simulink model "simL0_multiPath"  (R2024a)
settings: Solver=ode4  StartTime=0.0  StopTime=1500  FixedStep=0.01  MaxStep=0.01  MinStep=10^-3  RelTol=0.01
values from neighbouring files (symbols this model uses):
  MegAWESkite = yaml.ReadYaml('MegAWESkite.yaml',false,true)    [runMain.m]
undefined symbols (not defined in the file or in its folder): actuatorLimit, controllerGains_retraction, controllerGains_traction, DiscIntNeverNeededParam, ENVMT, pathparam, simInit, tetherParams, winchParameter
libraries: simulink x9, slpidlib x9, sharedtransform x3, aerolibutil x3, dspswit3 x2, dspinverses x2, shared6dof x1, simulink_extras x1, dspsigops x1, dspstat3 x1, vrlib x1
(part 2 of 5)

== system simL0_multiPath/GroundStationMegAWES/PureTorqueControl ==
  F_t_m_grnd : Inport
  F_t_set : Inport  Port=2
  theta_dot : Inport  Port=3
  Enable : EnablePort  StatesWhenEnabling=reset
  Constant4 : Constant  Value=winchParameter.a_max/winchParameter.radius
  Constant5 : Constant  Value=winchParameter.a_min/winchParameter.radius
  Dot Product1 : DotProduct  OutDataTypeStr=Inherit: Inherit via internal rule
  FT set : Scope  NumInputPorts=2
  Gain : Gain  Gain=winchParameter.inertia
  Gain1 : Gain  Gain=winchParameter.inertia
  Gain2 : Gain  Gain=winchParameter.friction
  Gain4 : Gain  Gain=winchParameter.radius
  PID Controller : slpidlib/PID Controller  Controller=PI  Form=Parallel  TimeDomain=Continuous-time  UseExternalTs=off  SampleTime=-1  IntegratorMethod=Forward Euler  FilterMethod=Forward Euler  ControllerParametersSource=internal  P=winchParameter.kp  I=winchParameter.ki  UseKiTs=off  D=0  UseExternalDerivativeSource=off  N=100  UseFilter=on  TunerSelectOption=Transfer Function Based (PID Tuner App)  InitialConditionSource=internal  InitialConditionForIntegrator=0  InitialConditionForFilter=0  DifferentiatorICPrevScaledInput=0  ExternalReset=none  TrackingMode=off  Kt=1  LimitOutput=off  SatLimitsSource=internal  UpperSaturationLimit=inf  LowerSaturationLimit=-inf  LinearizeAsGain=on  AntiWindupMode=none  Kb=1  LimitIntegrator=off  UpperIntegratorSaturationLimit=inf  LowerIntegratorSaturationLimit=-inf  POutMin=[]  POutMax=[]  IOutMin=[]  IOutMax=[]  DOutMin=[]  DOutMax=[]  NOutMin=[]  NOutMax=[]  SumOutMin=[]  SumOutMax=[]  SaturationOutMin=[]  SaturationOutMax=[]  PParamMin=[]  PParamMax=[]  IParamMin=[]  IParamMax=[]  DParamMin=[]  DParamMax=[]  NParamMin=[]  NParamMax=[]  KbParamMin=[]  KbParamMax=[]  KtParamMin=[]  KtParamMax=[]  KbOutMin=[]  KbOutMax=[]  KtOutMin=[]  KtOutMax=[]  IntegratorOutMin=[]  IntegratorOutMax=[]  FilterOutMin=[]  FilterOutMax=[]  SumI1OutMin=[]  SumI1OutMax=[]  SumI2OutMin=[]  SumI2OutMax=[]  SumI3OutMin=[]  SumI3OutMax=[]  SumI4OutMin=[]  SumI4OutMax=[]  SumDOutMin=[]  SumDOutMax=[]  DifferentiatorOutMin=[]  DifferentiatorOutMax=[]  FilterDiffOutCoefMin=[]  FilterDiffOutCoefMax=[]  ReciprocalOutMin=[]  ReciprocalOutMax=[]  SumDenOutMin=[]  SumDenOutMax=[]  SumNumOutMin=[]  SumNumOutMax=[]  DivideOutMin=[]  DivideOutMax=[]  UdiffTsProdOutMin=[]  UdiffTsProdOutMax=[]  NTsProdOutMin=[]  NTsProdOutMax=[]  UintegralTsProdOutMin=[]  UintegralTsProdOutMax=[]  UngainTsProdOutMin=[]  UngainTsProdOutMax=[]  ClampingZeroOutDataTypeStr=Inherit: Inherit via back propagation  ClampingZeroOutMin=[]  ClampingZeroOutMax=[]  FilterDenConstantOutDataTypeStr=Inherit: Inherit via back propagation  FilterDenConstantOutMin=[]  FilterDenConstantOutMax=[]  PCopyOutDataTypeStr=Inherit: Inherit via back propagation  PCopyOutMin=[]  PCopyOutMax=[]  NCopyOutDataTypeStr=Inherit: Inherit via back propagation  NCopyOutMin=[]  NCopyOutMax=[]  IntegratorContinuousStateAttributes=''  IntegratorStateMustResolveToSignalObject=off  IntegratorRTWStateStorageClass=Auto  FilterContinuousStateAttributes=''  FilterStateMustResolveToSignalObject=off  FilterRTWStateStorageClass=Auto  ParallelPVariant=InternalParameters  IdealPVariant=Disabled  IVariant=InternalParameters  DVariant=Disabled  IntegratorVariant=Continuous  SatVariant=Disabled  AWVariant=Passthrough  PCopyVariant=Disabled  TRVariant=Disabled  FdbkBlocksVariant=Forward  IdealPFdbkVariant=Disabled  SatFdbkVariant=Disabled  DerivativeFilterVariant=Disabled  NVariant=Disabled  NCopyVariant=Disabled_SignalSpec  FilterICVariant=Disabled  IntegratorICVariant=InternalICs  ExternalResetVariant=Disabled  TRSumVariant=Passthrough  SumFdbkVariant=Disabled  SumVariant=Sum_PI  TsampFilterVariant=InternalTs  TsampNgainVariant=Passthrough  TsampIntegralVariant=Disabled_SignalSpec  ExternalSaturationOutDataTypeStr=Inherit: Same as second input  DerivativeSourceVariant=Disabled
  Saturation Dynamic : simulink/Discontinuities/Saturation Dynamic  OutMin=[]  OutMax=[]  OutDataTypeStr=Inherit: Same as second input  OutDataType=fixdt(1, 16)  OutScaling=2^-10  DoSatur=off
  Sqrt1 : Sqrt
  Sum2 : Sum  Inputs=-++
  Sum4 : Sum  Inputs=-++
  Sum6 : Sum  Inputs=|-+
  torque_cmd : Outport  VectorParamsAs1DForOutWhenUnconnected=off
  wires:
  Sqrt1/1 -> FT set/1, Sum6/2
  F_t_set/1 -> FT set/2, Sum6/1
  Gain4/1 -> Sum2/1, Sum4/1
  Constant4/1 -> Gain/1
  Gain/1 -> Sum2/2
  Sum2/1 -> Saturation Dynamic/1
  Constant5/1 -> Gain1/1
  Gain1/1 -> Sum4/2
  Sum4/1 -> Saturation Dynamic/3
  Gain2/1 -> Sum4/3, Sum2/3
  Dot Product1/1 -> Sqrt1/1
  F_t_m_grnd/1 -> Dot Product1/1, Dot Product1/2, Gain4/1
  theta_dot/1 -> Gain2/1
  Sum6/1 -> PID Controller/1
  Saturation Dynamic/1 -> torque_cmd/1
  PID Controller/1 -> Saturation Dynamic/2

== system simL0_multiPath/GroundStationMegAWES/Traction winch controller ==
  v_ro : Inport
  Ft_ground_W : Inport  Port=2
  Calculate Ft_ref : Subsystem
  MegAWES convention is that a positive torque leads to reel-out : Gain  Gain=-1
  Sum : Sum  Inputs=|+-
  feedforward : Gain  Gain=winchParameter.radius
  reel-out : Scope
  tether force : Scope  NumInputPorts=3
  torque : Scope
  traction_torque_cmd : Outport
  Ft_ref : Outport  Port=2
  Ft_ground : Outport  Port=3
  wires:
  v_ro/1 -> reel-out/1, Calculate Ft_ref/1(v_ro)
  Ft_ground_W/1 -> Ft_ground/1, Sum/2, tether force/2
  Sum/1 -> tether force/3
  feedforward/1 -> MegAWES convention is that a positive torque leads to reel-out/1, torque/1  "torque_md_tot"
  MegAWES convention is that a positive torque leads to reel-out/1 -> traction_torque_cmd/1
  Calculate Ft_ref/1(Ft_ref) -> feedforward/1, Ft_ref/1, tether force/1, Sum/1

== system simL0_multiPath/GroundStationMegAWES/WinchDynamics ==
  for_tether_tot : Inport
  control_moments : Inport  Port=2
  Discrete-Time Integrator : DiscreteIntegrator  InitialCondition=winchParameter.lj_dot_init  SampleTime=-1  LimitOutput=on  UpperSaturationLimit=winchParameter.v_max/winchParameter.radius  LowerSaturationLimit=winchParameter.v_min/winchParameter.radius  ICPrevOutput=DiscIntNeverNeededParam  ICPrevScaledInput=DiscIntNeverNeededParam
  Gain{,2..6} (6 alike) : Gain  Gain=winchParameter.radius
  Gain1 : Gain  Gain=1/winchParameter.inertia
  Gain7 : Gain  Gain=winchParameter.friction
  Integrator : Integrator  InitialCondition=tetherParams.tether_inital_lenght/winchParameter.radius
  Saturation1 : Saturate  UpperLimit=winchParameter.a_max/winchParameter.radius  LowerLimit=winchParameter.a_min/winchParameter.radius
  Sum : Sum  Inputs=+-+
  winch acc : Scope  NumInputPorts=2
  tether_length : Outport  VectorParamsAs1DForOutWhenUnconnected=off
  theta_dot : Outport  Port=2  VectorParamsAs1DForOutWhenUnconnected=off
  winch_acc : Outport  Port=3  VectorParamsAs1DForOutWhenUnconnected=off
  winch_vel : Outport  Port=4  VectorParamsAs1DForOutWhenUnconnected=off
  wires:
  Gain/1 -> tether_length/1
  Gain2/1 -> Sum/1
  Sum/1 -> Gain1/1
  Integrator/1 -> Gain/1  "winch_angle"
  Discrete-Time Integrator/1 -> Gain4/1, Gain7/1, theta_dot/1, Integrator/1  "winch_angVel"
  control_moments/1 -> Sum/3
  Gain7/1 -> Sum/2
  for_tether_tot/1 -> Gain2/1
  Gain1/1 -> Saturation1/1, Gain5/1, Gain3/1
  Saturation1/1 -> Discrete-Time Integrator/1, Gain6/1  "omega_dot"
  Gain4/1 -> winch_vel/1
  Gain3/1 -> winch_acc/1
  Gain5/1 -> winch acc/1
  Gain6/1 -> winch acc/2

== system simL0_multiPath/Output/Convergence_check ==
  P_mech : Inport
  flightMode : Inport  Port=2
  AND : Logic  AllPortsSameDT=off  OutDataTypeStr=boolean
  Compare To Constant1 : simulink/Logic and Bit Operations/Compare To Constant  relop=>=  const=simInit.numCyclesMinimumConv  OutDataTypeStr=boolean
  Constant1 : Constant  Value=simInit.thresholdConv_power/simInit.numCyclesMinimumConv
  Delay{1..4,6..7} (6 alike) : Delay  DelayLength=1  InitialCondition=0
  Delay5 : Delay  DelayLength=1  InitialCondition=simInit.thresholdConv_power+1000
  MATLAB Function2 : MATLAB Function  TreatAsAtomicUnit=on
  Matrix Multiply : Product
  Relational Operator1 : RelationalOperator  Operator=<=  OutDataTypeStr=boolean  RndMeth=Simplest  InputSameDT=off
  Scope : Scope
  Scope1 : Scope
  Stop Simulation : Stop
  power_conv_flag : Outport  VectorParamsAs1DForOutWhenUnconnected=off
  error_power : Outport  Port=2  VectorParamsAs1DForOutWhenUnconnected=off
  No_cycles : Outport  Port=3
  cycle_signal_counter : Outport  Port=4  VectorParamsAs1DForOutWhenUnconnected=off
  wires:
  Delay5/1 -> MATLAB Function2/7(e_old)
  Constant1/1 -> Matrix Multiply/1
  Matrix Multiply/1 -> Relational Operator1/2
  Compare To Constant1/1 -> AND/2
  flightMode/1 -> Scope1/1, MATLAB Function2/6(flightMode)
  Delay7/1 -> MATLAB Function2/8("cnt_max_mat ")
  MATLAB Function2/4(cnt) -> Delay1/1
  Delay4/1 -> MATLAB Function2/1("flag ")
  Delay3/1 -> MATLAB Function2/3("p_sum ")
  Relational Operator1/1 -> AND/1
  Delay1/1 -> MATLAB Function2/4("cnt ")
  MATLAB Function2/3(p_sum) -> Delay3/1
  MATLAB Function2/1(flag) -> Delay4/1
  Delay2/1 -> MATLAB Function2/2(m_old)
  MATLAB Function2/7(cycles_cnt) -> Delay6/1, No_cycles/1, Matrix Multiply/2, Compare To Constant1/1, Scope/1
  MATLAB Function2/2(m_new) -> Delay2/1
  AND/1 -> power_conv_flag/1, Stop Simulation/1
  P_mech/1 -> MATLAB Function2/5(u)
  Delay6/1 -> MATLAB Function2/9("cycles_cnt ")
  MATLAB Function2/6(cnt_max_mat) -> cycle_signal_counter/1, Delay7/1
  MATLAB Function2/5(e_new) -> Delay5/1, error_power/1, Relational Operator1/1

== system simL0_multiPath/aerodynamic forces/HLW ==
  In1 : Inport
  Switch Solver Compiled : MATLAB Function  TreatAsAtomicUnit=on
  Out1 : Outport  VectorParamsAs1DForOutWhenUnconnected=off
  wires:
  Switch Solver Compiled/1(out) -> Out1/1
  In1/1 -> Switch Solver Compiled/1(input)

== system simL0_multiPath/aerodynamic forces/Lookup Tables ==
  Inputs : Inport
  Switch Solver Compiled : MATLAB Function  TreatAsAtomicUnit=on
  ForceMoment : Outport  VectorParamsAs1DForOutWhenUnconnected=off
  wires:
  Switch Solver Compiled/1(out) -> ForceMoment/1
  Inputs/1 -> Switch Solver Compiled/1(input)

== system simL0_multiPath/aerodynamic forces/SLW ==
  In1 : Inport
  Switch Solver Compiled : MATLAB Function  TreatAsAtomicUnit=on
  Out1 : Outport  VectorParamsAs1DForOutWhenUnconnected=off
  wires:
  Switch Solver Compiled/1(out) -> Out1/1
  In1/1 -> Switch Solver Compiled/1(input)

== system simL0_multiPath/aerodynamic forces/Subsystem ==
  In1 : Inport
  Demux5 : Demux  Outputs=10
  Mux : Mux  Inputs=8
  Mux1 : Mux  Inputs=2
  Out1 : Outport  VectorParamsAs1DForOutWhenUnconnected=off
  Out2 : Outport  Port=2  VectorParamsAs1DForOutWhenUnconnected=off
  wires:
  Demux5/3 -> Mux/3
  Demux5/7 -> Mux/7
  In1/1 -> Demux5/1
  Demux5/1 -> Mux/1
  Demux5/4 -> Mux/4
  Mux/1 -> Out1/1
  Demux5/5 -> Mux/5
  Demux5/6 -> Mux/6
  Demux5/8 -> Mux/8
  Demux5/9 -> Mux1/1
  Demux5/2 -> Mux/2
  Demux5/10 -> Mux1/2
  Mux1/1 -> Out2/1

== system simL0_multiPath/aerodynamic forces/Subsystem1 ==
  note: OLD
  note: increases the flap angle on the side, towards which the plane is rolling
  In1 : Inport
  Gain1 : Gain  Commented=on  Gain=-1.5
  Gain2 : Gain  Commented=on  Gain=-1
  Gain4 : Gain  Commented=on
  Gain5 : Gain  Commented=on  Gain=1.5
  Gain6 : Gain  Gain=-1
  Gain7 : Gain
  Switch : Switch  Commented=on  Criteria=u2 > Threshold  SaturateOnIntegerOverflow=off  InputSameDT=off
  Switch1 : Switch  Commented=on  Criteria=u2 > Threshold  SaturateOnIntegerOverflow=off  InputSameDT=off
  left flap : Outport  VectorParamsAs1DForOutWhenUnconnected=off
  right flap : Outport  Port=2  VectorParamsAs1DForOutWhenUnconnected=off
  wires:
  Gain1/1 -> Switch/1
  Gain2/1 -> Switch/3
  Gain4/1 -> Switch1/1
  Gain5/1 -> Switch1/3
  Gain6/1 -> right flap/1
  Gain7/1 -> left flap/1
  In1/1 -> Gain4/1, Switch1/2, Gain5/1, Gain2/1, Switch/2, Gain1/1, Gain6/1, Gain7/1

== system simL0_multiPath/Controls/ FlightControl/Angle_of_Attack ==
  desired_descent_angle : Inport
  flightState : Inport  Port=2
  Constant12 : Constant  Value=MegAWESkite.MainWing.alphaMax
  Degrees to Radians : simulink_extras/Transformations/Degrees to Radians
  Multiply : Gain  Gain=0.75
  Multiport Switch3 : MultiPortSwitch  DiagnosticForDefault=None  SaturateOnIntegerOverflow=off  InputSameDT=off
  desired_alpha : Outport
  wires:
  desired_descent_angle/1 -> Multiport Switch3/4, Multiport Switch3/3
  Degrees to Radians/1 -> Multiport Switch3/2
  flightState/1 -> Multiport Switch3/1
  Constant12/1 -> Multiply/1
  Multiply/1 -> Degrees to Radians/1
  Multiport Switch3/1 -> desired_alpha/1

== system simL0_multiPath/Controls/ FlightControl/Convert YPR-e_to_tan ==
  kite_pos : Inport
  kite_angles : Inport  Port=2
  Convert YPR-etotan : MATLAB Function  TreatAsAtomicUnit=on
  Demux8 : Demux  Outputs=3
  Demux9 : Demux  Outputs=3
  Mux5 : Mux  Inputs=6
  Scope15 : Scope
  roll_tang : Outport
  pitch_tang : Outport  Port=2
  yaw_tang : Outport  Port=3
  actual_roll : Outport  Port=4
  wires:
  Demux8/2 -> Mux5/2
  Demux9/3 -> Mux5/6
  Convert YPR-etotan/2(a_pitch) -> pitch_tang/1
  Demux8/3 -> Mux5/3
  Demux9/2 -> Mux5/5
  Convert YPR-etotan/1(a_roll) -> Scope15/1, roll_tang/1
  Convert YPR-etotan/3(a_yaw) -> yaw_tang/1
  Demux8/1 -> Mux5/1
  Mux5/1 -> Convert YPR-etotan/1(input)
  kite_angles/1 -> Demux9/1
  Demux9/1 -> actual_roll/1, Mux5/4
  kite_pos/1 -> Demux8/1

== system simL0_multiPath/Controls/ FlightControl/EarthtoWind ==
  E_vec : Inport
  Demux : Demux  Outputs=3
  Gain : Gain
  Gain1 : Gain  Gain=-1
  Gain2 : Gain  Gain=-1
  Mux4 : Mux  Inputs=3
  W_vec : Outport
  wires:
  Demux/2 -> Gain1/1
  Demux/1 -> Gain/1
  Gain1/1 -> Mux4/2
  Gain/1 -> Mux4/1
  Gain2/1 -> Mux4/3
  E_vec/1 -> Demux/1
  Mux4/1 -> W_vec/1
  Demux/3 -> Gain2/1

== system simL0_multiPath/Controls/ FlightControl/EarthtoWind1 ==
  E_vec : Inport
  Demux : Demux  Outputs=3
  Gain : Gain
  Gain1 : Gain  Gain=-1
  Gain2 : Gain  Gain=-1
  Mux4 : Mux  Inputs=3
  W_vec : Outport
  wires:
  Demux/2 -> Gain1/1
  Demux/1 -> Gain/1
  Gain1/1 -> Mux4/2
  Gain/1 -> Mux4/1
  Gain2/1 -> Mux4/3
  E_vec/1 -> Demux/1
  Mux4/1 -> W_vec/1
  Demux/3 -> Gain2/1

== system simL0_multiPath/Controls/ FlightControl/EarthtoWind2 ==
  E_vec : Inport
  Demux : Demux  Outputs=3
  Gain : Gain
  Gain1 : Gain  Gain=-1
  Gain2 : Gain  Gain=-1
  Mux4 : Mux  Inputs=3
  W_vec : Outport
  wires:
  Demux/2 -> Gain1/1
  Demux/1 -> Gain/1
  Gain1/1 -> Mux4/2
  Gain/1 -> Mux4/1
  Gain2/1 -> Mux4/3
  E_vec/1 -> Demux/1
  Mux4/1 -> W_vec/1
  Demux/3 -> Gain2/1

== system simL0_multiPath/Controls/ FlightControl/EarthtoWind3 ==
  E_vec : Inport
  Demux : Demux  Outputs=3
  Gain : Gain
  Gain1 : Gain  Gain=-1
  Gain2 : Gain  Gain=-1
  Mux4 : Mux  Inputs=3
  W_vec : Outport
  wires:
  Demux/2 -> Gain1/1
  Demux/1 -> Gain/1
  Gain1/1 -> Mux4/2
  Gain/1 -> Mux4/1
  Gain2/1 -> Mux4/3
  E_vec/1 -> Demux/1
  Mux4/1 -> W_vec/1
  Demux/3 -> Gain2/1

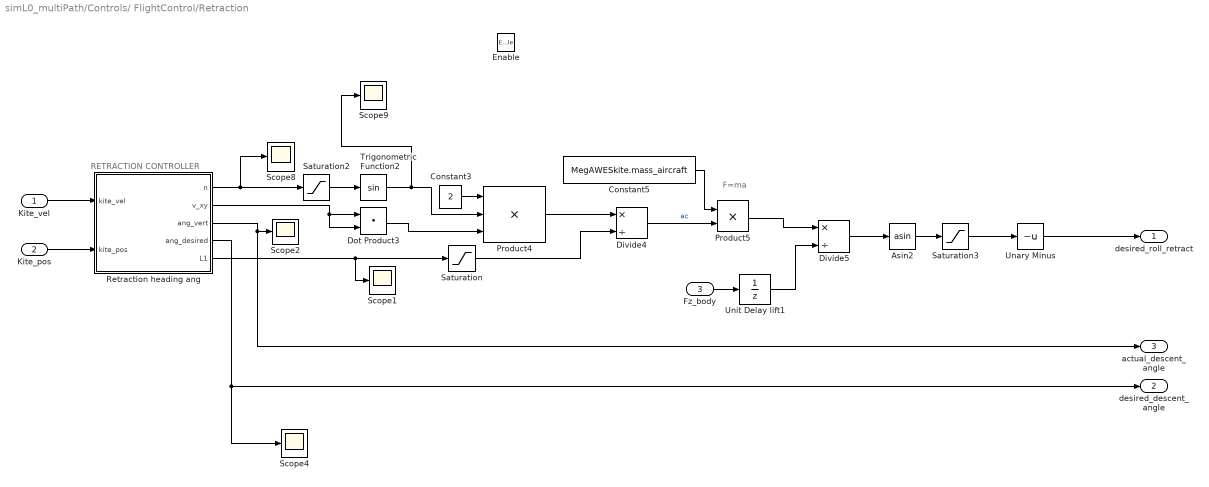
== system simL0_multiPath/Controls/ FlightControl/Retraction ==
  note: F=ma
  note: RETRACTION CONTROLLER
  Kite_vel : Inport
  Kite_pos : Inport  Port=2
  Fz_body : Inport  Port=3
  Enable : EnablePort  StatesWhenEnabling=reset
  Asin2 : Trigonometry  Operator=asin
  Constant3 : Constant  Value=2
  Constant5 : Constant  Value=MegAWESkite.mass_aircraft
  Divide4 : Product  Inputs=*/
  Divide5 : Product  Inputs=*/
  Dot Product3 : DotProduct  OutDataTypeStr=Inherit: Inherit via internal rule
  Product4 : Product  Inputs=3
  Product5 : Product
  Retraction heading ang : MATLAB Function  TreatAsAtomicUnit=on
  Saturation : Saturate  UpperLimit=inf  LowerLimit=100
  Saturation2 : Saturate  UpperLimit=pi/2  LowerLimit=-pi/2
  Saturation3 : Saturate  UpperLimit=1  LowerLimit=-1
  Scope{1..2,4,8..9} (5 alike) : Scope
  Trigonometric Function2 : Trigonometry
  Unary Minus : UnaryMinus
  Unit Delay lift1 : UnitDelay  InitialCondition=1  SampleTime=-1  HasFrameUpgradeWarning=on
  desired_roll_retract : Outport
  desired_descent_angle : Outport  Port=2
  actual_descent_angle : Outport  Port=3
  wires:
  Saturation3/1 -> Unary Minus/1
  Retraction heading ang/3(ang_vert) -> actual_descent_angle/1, Scope2/1
  Retraction heading ang/1(n) -> Scope8/1, Saturation2/1
  Fz_body/1 -> Unit Delay lift1/1
  Product4/1 -> Divide4/1
  Retraction heading ang/2(v_xy) -> Dot Product3/2, Dot Product3/1
  Divide4/1 -> Product5/2  "ac"
  Retraction heading ang/4(ang_desired) -> desired_descent_angle/1, Scope4/1
  Unary Minus/1 -> desired_roll_retract/1
  Divide5/1 -> Asin2/1
  Constant3/1 -> Product4/1
  Dot Product3/1 -> Product4/3
  Kite_vel/1 -> Retraction heading ang/1(kite_vel)
  Asin2/1 -> Saturation3/1
  Trigonometric Function2/1 -> Scope9/1, Product4/2
  Kite_pos/1 -> Retraction heading ang/2(kite_pos)
  Product5/1 -> Divide5/1
  Unit Delay lift1/1 -> Divide5/2
  Saturation2/1 -> Trigonometric Function2/1
  Constant5/1 -> Product5/1
  Retraction heading ang/5(L1) -> Scope1/1, Saturation/1
  Saturation/1 -> Divide4/2

== system simL0_multiPath/Controls/ FlightControl/Switch_flystate ==
  s_path : Inport
  Counter1 : dspswit3/Counter  Direction=Up  CountEvent=Rising edge  CounterSize=User defined  MaxCount=255  InitialCount=0  Output=Count  HitValue=32  ResetInput=off  SamplesPerFrame=1  Ts=1  CntDtype=double  HitDtype=Logical
  MATLAB Function : MATLAB Function  TreatAsAtomicUnit=on
  Zero Crossing : dspsigops/Zero Crossing  InputProcessing=Columns as channels (frame based)
  n_cycle : Outport
  pos_cond : Outport  Port=2
  trans_flag : Outport  Port=3
  wires:
  Counter1/1 -> n_cycle/1
  s_path/1 -> MATLAB Function/1(s)
  Zero Crossing/1 -> Counter1/1
  MATLAB Function/1(r) -> pos_cond/1, Zero Crossing/1
  MATLAB Function/2(t) -> trans_flag/1

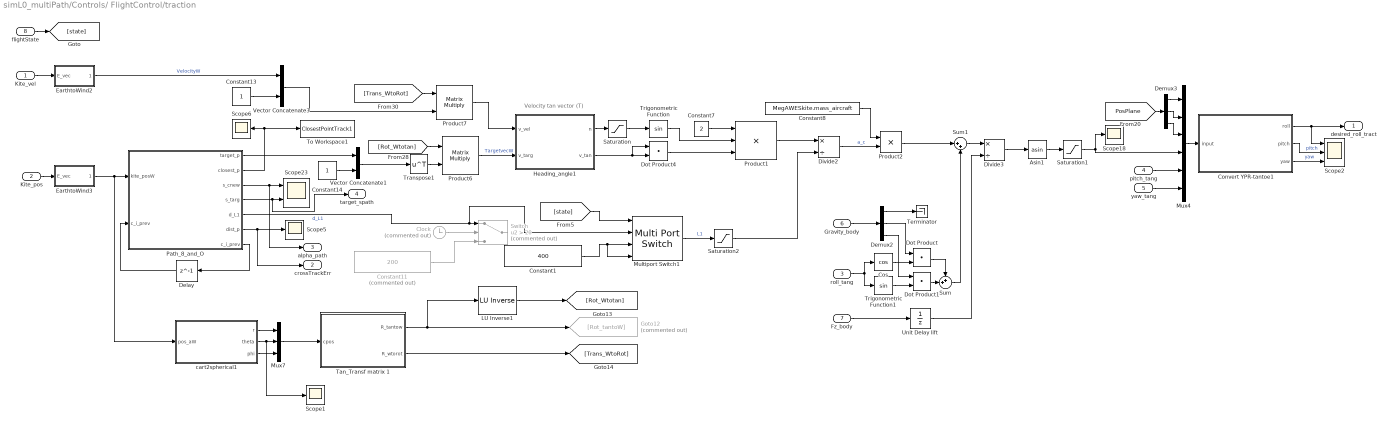
== system simL0_multiPath/Controls/ FlightControl/traction ==
  note: Velocity tan vector (T)
  Kite_vel : Inport
  Kite_pos : Inport  Port=2
  roll_tang : Inport  Port=3
  pitch_tang : Inport  Port=4
  yaw_tang : Inport  Port=5
  Gravity_body : Inport  Port=6
  Fz_body : Inport  Port=7
  flightState : Inport  Port=8
  " LU Inverse1" : dspinverses/ LU Inverse
  Asin1 : Trigonometry  Operator=asin
  Clock : Clock  Commented=on
  Constant1 : Constant  Value=400
  Constant11 : Constant  Commented=on  Value=200
  Constant13 : Constant
  Constant14 : Constant
  Constant7 : Constant  Value=2
  Constant8 : Constant  Value=MegAWESkite.mass_aircraft
  Convert YPR-tantoe1 : MATLAB Function  TreatAsAtomicUnit=on
  Cos : Trigonometry  Operator=cos
  Delay : Delay  DelayLength=1  InitialCondition=25
  Demux2 : Demux  Outputs=3
  Demux3 : Demux  Outputs=3
  Divide2 : Product  Inputs=*/
  Divide3 : Product  Inputs=*/
  Dot Product : DotProduct  OutDataTypeStr=Inherit: Inherit via internal rule
  Dot Product1 : DotProduct  OutDataTypeStr=Inherit: Inherit via internal rule
  Dot Product4 : DotProduct  OutDataTypeStr=Inherit: Inherit via internal rule
  EarthtoWind2 : Subsystem
  EarthtoWind3 : Subsystem
  Goto12 : Goto  Commented=on  GotoTag=Rot_tantoW
  Heading_angle1 : MATLAB Function  TreatAsAtomicUnit=on
  Multiport Switch1 : MultiPortSwitch  DiagnosticForDefault=None  SaturateOnIntegerOverflow=off  InputSameDT=off
  Mux4 : Mux  Inputs=6
  Mux7 : Mux  Inputs=3
  Path_8_and_O : MATLAB Function  TreatAsAtomicUnit=on
  Product1 : Product  Inputs=3
  Product2 : Product
  Product6 : Product  Multiplication=Matrix(*)
  Product7 : Product  Multiplication=Matrix(*)
  Saturation : Saturate  UpperLimit=pi/4  LowerLimit=-pi/4
  Saturation1 : Saturate  UpperLimit=1  LowerLimit=-1
  Saturation2 : Saturate  UpperLimit=inf  LowerLimit=50
  Scope{1,5..6,18} (4 alike) : Scope
  Scope2 : Scope  NumInputPorts=3
  Scope23 : Scope  NumInputPorts=2
  Sum : Sum  Inputs=++|
  Sum1 : Sum  Inputs=|++
  Switch : Switch  Commented=on  Criteria=u2 > Threshold  Threshold=20  SaturateOnIntegerOverflow=off  InputSameDT=off
  Tan_Transf matrix 1 : MATLAB Function  TreatAsAtomicUnit=on
  Terminator : Terminator
  To Workspace1 : ToWorkspace  VariableName=ClosestPointTrack1  SaveFormat=Timeseries  SampleTime=-1
  Transpose1 : Math  Operator=transpose
  Trigonometric Function : Trigonometry
  Trigonometric Function1 : Trigonometry
  Unit Delay lift : UnitDelay  InitialCondition=1  SampleTime=-1  HasFrameUpgradeWarning=on
  Vector Concatenate1 : Concatenate
  Vector Concatenate3 : Concatenate
  cart2spherical1 : MATLAB Function  TreatAsAtomicUnit=on
  desired_roll_tract : Outport
  crossTrackErr : Outport  Port=2
  alpha_path : Outport  Port=3
  target_spath : Outport  Port=4
  wires:
  Demux2/3 -> Dot Product1/1
  Constant13/1 -> Vector Concatenate3/2
  Convert YPR-tantoe1/3(yaw) -> Scope2/3  "yaw"
  Heading_angle1/2(v_tan) -> Dot Product4/1, Dot Product4/2
  Dot Product/1 -> Sum/1
  Constant8/1 -> Product2/1
  Convert YPR-tantoe1/1(roll) -> desired_roll_tract/1, Scope2/1
  Trigonometric Function/1 -> Product1/2
  Path_8_and_O/3(s_cnew) -> alpha_path/1, Scope23/1
  Path_8_and_O/4(s_targ) -> target_spath/1, Scope23/2
  Product7/1 -> Heading_angle1/1(v_vel)
  Demux3/3 -> Mux4/3
  Saturation/1 -> Trigonometric Function/1
  Dot Product1/1 -> Sum/2
  Demux3/2 -> Mux4/2
  Divide2/1 -> Product2/2  "a_c"
  Product2/1 -> Sum1/1
  Cos/1 -> Dot Product/2
  Divide3/1 -> Asin1/1
  Constant7/1 -> Product1/1
  Asin1/1 -> Saturation1/1
  Gravity_body/1 -> Demux2/1
  Product1/1 -> Divide2/1
  Heading_angle1/1(n) -> Saturation/1
  Unit Delay lift/1 -> Divide3/2
  Path_8_and_O/6(dist_p) -> crossTrackErr/1, Scope5/1
  Sum/1 -> Sum1/2
  EarthtoWind2/1(W_vec) -> Vector Concatenate3/1  "VelocityW"
  Convert YPR-tantoe1/2(pitch) -> Scope2/2  "pitch"
  Saturation1/1 -> Scope18/1, Mux4/4
  [state] -> Multiport Switch1/1
  Mux4/1 -> Convert YPR-tantoe1/1(input)
  Demux3/1 -> Mux4/1
  Trigonometric Function1/1 -> Dot Product1/2
  Demux2/1 -> Terminator/1
  Fz_body/1 -> Unit Delay lift/1
  Multiport Switch1/1 -> Saturation2/1  "L1"
  Vector Concatenate3/1 -> Product7/2
  [Trans_WtoRot] -> Product7/1
  Demux2/2 -> Dot Product/1
  [PosPlane] -> Demux3/1
  pitch_tang/1 -> Mux4/5
  [Rot_Wtotan] -> Product6/1
  Constant14/1 -> Vector Concatenate1/2
  Transpose1/1 -> Product6/2
  Kite_pos/1 -> EarthtoWind3/1(E_vec)
  Product6/1 -> Heading_angle1/2(v_targ)  "TargetvecW"
  Sum1/1 -> Divide3/1
  Dot Product4/1 -> Product1/3
  Path_8_and_O/1(target_p) -> Vector Concatenate1/1
  yaw_tang/1 -> Mux4/6
  Vector Concatenate1/1 -> Transpose1/1
  Path_8_and_O/5(d_L1) -> Multiport Switch1/2, Switch/1  "d_L1"
  roll_tang/1 -> Trigonometric Function1/1, Cos/1
  Path_8_and_O/2(closest_p) -> To Workspace1/1, Scope6/1
  Kite_vel/1 -> EarthtoWind2/1(E_vec)
  " LU Inverse1"/1 -> [Rot_Wtotan]
  Mux7/1 -> Tan_Transf matrix 1/1(cpos)
  Tan_Transf matrix 1/1(R_tantow) -> Goto12/1, " LU Inverse1"/1
  cart2spherical1/1(r) -> Mux7/1
  cart2spherical1/3(phi) -> Mux7/3
  Tan_Transf matrix 1/2(R_wtorot) -> [Trans_WtoRot]
  EarthtoWind3/1(W_vec) -> cart2spherical1/1(pos_aW), Path_8_and_O/1(kite_posW)
  cart2spherical1/2(theta) -> Scope1/1, Mux7/2
  flightState/1 -> [state]
  Path_8_and_O/7(c_i_prev) -> Delay/1
  Delay/1 -> Path_8_and_O/2("c_i_prev ")
  Saturation2/1 -> Divide2/2
  Constant11/1 -> Switch/3
  Clock/1 -> Switch/2
  Constant1/1 -> Multiport Switch1/4, Multiport Switch1/3

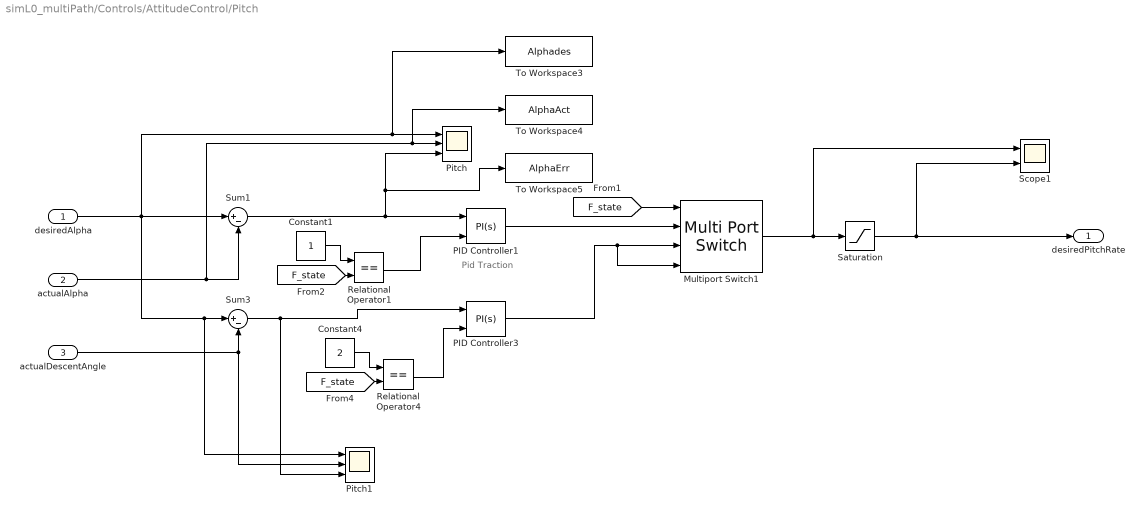
== system simL0_multiPath/Controls/AttitudeControl/Pitch ==
  note: Pid Traction
  desiredAlpha : Inport
  actualAlpha : Inport  Port=2
  actualDescentAngle : Inport  Port=3
  Constant1 : Constant
  Constant4 : Constant  Value=2
  Multiport Switch1 : MultiPortSwitch  DiagnosticForDefault=None  SaturateOnIntegerOverflow=off  InputSameDT=off
  PID Controller1 : slpidlib/PID Controller  Controller=PI  Form=Parallel  TimeDomain=Continuous-time  UseExternalTs=off  SampleTime=-1  IntegratorMethod=Forward Euler  FilterMethod=Forward Euler  ControllerParametersSource=internal  P=controllerGains_traction.attitudePitch_P  I=controllerGains_traction.attitudePitch_I  UseKiTs=off  D=0  UseExternalDerivativeSource=off  N=1  UseFilter=on  TunerSelectOption=Transfer Function Based (PID Tuner App)  InitialConditionSource=internal  InitialConditionForIntegrator=0  InitialConditionForFilter=0  DifferentiatorICPrevScaledInput=0  ExternalReset=rising  TrackingMode=off  Kt=1  LimitOutput=off  SatLimitsSource=internal  UpperSaturationLimit=pi  LowerSaturationLimit=-pi  LinearizeAsGain=on  AntiWindupMode=none  Kb=50  LimitIntegrator=off  UpperIntegratorSaturationLimit=inf  LowerIntegratorSaturationLimit=-inf  POutMin=[]  POutMax=[]  IOutMin=[]  IOutMax=[]  DOutMin=[]  DOutMax=[]  NOutMin=[]  NOutMax=[]  SumOutMin=[]  SumOutMax=[]  SaturationOutMin=[]  SaturationOutMax=[]  PParamMin=[]  PParamMax=[]  IParamMin=[]  IParamMax=[]  DParamMin=[]  DParamMax=[]  NParamMin=[]  NParamMax=[]  KbParamMin=[]  KbParamMax=[]  KtParamMin=[]  KtParamMax=[]  KbOutMin=[]  KbOutMax=[]  KtOutMin=[]  KtOutMax=[]  IntegratorOutMin=[]  IntegratorOutMax=[]  FilterOutMin=[]  FilterOutMax=[]  SumI1OutMin=[]  SumI1OutMax=[]  SumI2OutMin=[]  SumI2OutMax=[]  SumI3OutMin=[]  SumI3OutMax=[]  SumI4OutMin=[]  SumI4OutMax=[]  SumDOutMin=[]  SumDOutMax=[]  DifferentiatorOutMin=[]  DifferentiatorOutMax=[]  FilterDiffOutCoefMin=[]  FilterDiffOutCoefMax=[]  ReciprocalOutMin=[]  ReciprocalOutMax=[]  SumDenOutMin=[]  SumDenOutMax=[]  SumNumOutMin=[]  SumNumOutMax=[]  DivideOutMin=[]  DivideOutMax=[]  UdiffTsProdOutMin=[]  UdiffTsProdOutMax=[]  NTsProdOutMin=[]  NTsProdOutMax=[]  UintegralTsProdOutMin=[]  UintegralTsProdOutMax=[]  UngainTsProdOutMin=[]  UngainTsProdOutMax=[]  ClampingZeroOutDataTypeStr=Inherit: Inherit via back propagation  ClampingZeroOutMin=[]  ClampingZeroOutMax=[]  FilterDenConstantOutDataTypeStr=Inherit: Inherit via back propagation  FilterDenConstantOutMin=[]  FilterDenConstantOutMax=[]  PCopyOutDataTypeStr=Inherit: Inherit via back propagation  PCopyOutMin=[]  PCopyOutMax=[]  NCopyOutDataTypeStr=Inherit: Inherit via back propagation  NCopyOutMin=[]  NCopyOutMax=[]  IntegratorContinuousStateAttributes=''  IntegratorStateMustResolveToSignalObject=off  IntegratorRTWStateStorageClass=Auto  FilterContinuousStateAttributes=''  FilterStateMustResolveToSignalObject=off  FilterRTWStateStorageClass=Auto  ParallelPVariant=InternalParameters  IdealPVariant=Disabled  IVariant=InternalParameters  DVariant=Disabled  IntegratorVariant=Continuous  SatVariant=Disabled  AWVariant=Passthrough  PCopyVariant=Disabled  TRVariant=Disabled  FdbkBlocksVariant=Forward  IdealPFdbkVariant=Disabled  SatFdbkVariant=Disabled  DerivativeFilterVariant=Disabled  NVariant=Disabled  NCopyVariant=Disabled_SignalSpec  FilterICVariant=Disabled  IntegratorICVariant=InternalICs  ExternalResetVariant=ExternalReset  TRSumVariant=Passthrough  SumFdbkVariant=Disabled  SumVariant=Sum_PI  TsampFilterVariant=InternalTs  TsampNgainVariant=Passthrough  TsampIntegralVariant=Disabled_SignalSpec  ExternalSaturationOutDataTypeStr=Inherit: Same as second input  DerivativeSourceVariant=Disabled
  PID Controller3 : slpidlib/PID Controller  Controller=PI  Form=Parallel  TimeDomain=Continuous-time  UseExternalTs=off  SampleTime=-1  IntegratorMethod=Forward Euler  FilterMethod=Forward Euler  ControllerParametersSource=internal  P=controllerGains_retraction.attitudePitch_P  I=controllerGains_retraction.attitudePitch_I  UseKiTs=off  D=0  UseExternalDerivativeSource=off  N=1  UseFilter=on  TunerSelectOption=Transfer Function Based (PID Tuner App)  InitialConditionSource=internal  InitialConditionForIntegrator=0  InitialConditionForFilter=0  DifferentiatorICPrevScaledInput=0  ExternalReset=rising  TrackingMode=off  Kt=1  LimitOutput=off  SatLimitsSource=internal  UpperSaturationLimit=pi  LowerSaturationLimit=-pi  LinearizeAsGain=on  AntiWindupMode=none  Kb=50  LimitIntegrator=off  UpperIntegratorSaturationLimit=inf  LowerIntegratorSaturationLimit=-inf  POutMin=[]  POutMax=[]  IOutMin=[]  IOutMax=[]  DOutMin=[]  DOutMax=[]  NOutMin=[]  NOutMax=[]  SumOutMin=[]  SumOutMax=[]  SaturationOutMin=[]  SaturationOutMax=[]  PParamMin=[]  PParamMax=[]  IParamMin=[]  IParamMax=[]  DParamMin=[]  DParamMax=[]  NParamMin=[]  NParamMax=[]  KbParamMin=[]  KbParamMax=[]  KtParamMin=[]  KtParamMax=[]  KbOutMin=[]  KbOutMax=[]  KtOutMin=[]  KtOutMax=[]  IntegratorOutMin=[]  IntegratorOutMax=[]  FilterOutMin=[]  FilterOutMax=[]  SumI1OutMin=[]  SumI1OutMax=[]  SumI2OutMin=[]  SumI2OutMax=[]  SumI3OutMin=[]  SumI3OutMax=[]  SumI4OutMin=[]  SumI4OutMax=[]  SumDOutMin=[]  SumDOutMax=[]  DifferentiatorOutMin=[]  DifferentiatorOutMax=[]  FilterDiffOutCoefMin=[]  FilterDiffOutCoefMax=[]  ReciprocalOutMin=[]  ReciprocalOutMax=[]  SumDenOutMin=[]  SumDenOutMax=[]  SumNumOutMin=[]  SumNumOutMax=[]  DivideOutMin=[]  DivideOutMax=[]  UdiffTsProdOutMin=[]  UdiffTsProdOutMax=[]  NTsProdOutMin=[]  NTsProdOutMax=[]  UintegralTsProdOutMin=[]  UintegralTsProdOutMax=[]  UngainTsProdOutMin=[]  UngainTsProdOutMax=[]  ClampingZeroOutDataTypeStr=Inherit: Inherit via back propagation  ClampingZeroOutMin=[]  ClampingZeroOutMax=[]  FilterDenConstantOutDataTypeStr=Inherit: Inherit via back propagation  FilterDenConstantOutMin=[]  FilterDenConstantOutMax=[]  PCopyOutDataTypeStr=Inherit: Inherit via back propagation  PCopyOutMin=[]  PCopyOutMax=[]  NCopyOutDataTypeStr=Inherit: Inherit via back propagation  NCopyOutMin=[]  NCopyOutMax=[]  IntegratorContinuousStateAttributes=''  IntegratorStateMustResolveToSignalObject=off  IntegratorRTWStateStorageClass=Auto  FilterContinuousStateAttributes=''  FilterStateMustResolveToSignalObject=off  FilterRTWStateStorageClass=Auto  ParallelPVariant=InternalParameters  IdealPVariant=Disabled  IVariant=InternalParameters  DVariant=Disabled  IntegratorVariant=Continuous  SatVariant=Disabled  AWVariant=Passthrough  PCopyVariant=Disabled  TRVariant=Disabled  FdbkBlocksVariant=Forward  IdealPFdbkVariant=Disabled  SatFdbkVariant=Disabled  DerivativeFilterVariant=Disabled  NVariant=Disabled  NCopyVariant=Disabled_SignalSpec  FilterICVariant=Disabled  IntegratorICVariant=InternalICs  ExternalResetVariant=ExternalReset  TRSumVariant=Passthrough  SumFdbkVariant=Disabled  SumVariant=Sum_PI  TsampFilterVariant=InternalTs  TsampNgainVariant=Passthrough  TsampIntegralVariant=Disabled_SignalSpec  ExternalSaturationOutDataTypeStr=Inherit: Same as second input  DerivativeSourceVariant=Disabled
  Pitch : Scope  NumInputPorts=3
  Pitch1 : Scope  NumInputPorts=3
  Relational Operator1 : RelationalOperator  Operator===  OutDataTypeStr=boolean  RndMeth=Simplest  InputSameDT=off
  Relational Operator4 : RelationalOperator  Operator===  OutDataTypeStr=boolean  RndMeth=Simplest  InputSameDT=off
  Saturation : Saturate  UpperLimit=20  LowerLimit=-20
  Scope1 : Scope  NumInputPorts=2
  Sum1 : Sum  Inputs=|+-
  Sum3 : Sum  Inputs=|+-
  To Workspace3 : ToWorkspace  VariableName=Alphades  SaveFormat=Timeseries  SampleTime=-1
  To Workspace4 : ToWorkspace  VariableName=AlphaAct  SaveFormat=Timeseries  SampleTime=-1
  To Workspace5 : ToWorkspace  VariableName=AlphaErr  SaveFormat=Timeseries  SampleTime=-1
  desiredPitchRate : Outport
  wires:
  Relational Operator4/1 -> PID Controller3/2
  Sum1/1 -> Pitch/3, To Workspace5/1, PID Controller1/1
  PID Controller1/1 -> Multiport Switch1/2
  Sum3/1 -> Pitch1/3, PID Controller3/1
  actualDescentAngle/1 -> Pitch1/2, Sum3/2
  Multiport Switch1/1 -> Scope1/1, Saturation/1
  PID Controller3/1 -> Multiport Switch1/4, Multiport Switch1/3
  Saturation/1 -> desiredPitchRate/1, Scope1/2
  Constant1/1 -> Relational Operator1/1
  [F_state] -> Relational Operator4/2
  Relational Operator1/1 -> PID Controller1/2
  Constant4/1 -> Relational Operator4/1
  desiredAlpha/1 -> Pitch1/1, Sum3/1, Sum1/1, To Workspace3/1, Pitch/1
  actualAlpha/1 -> To Workspace4/1, Pitch/2, Sum1/2
  [F_state] -> Relational Operator1/2
  [F_state] -> Multiport Switch1/1

== system simL0_multiPath/Controls/AttitudeControl/Roll ==
  desiredRoll : Inport
  actualRoll : Inport  Port=2
  Constant2 : Constant  Value=2
  Constant3 : Constant
  Multiport Switch2 : MultiPortSwitch  DiagnosticForDefault=None  SaturateOnIntegerOverflow=off  InputSameDT=off
  PID Controller2 : slpidlib/PID Controller  Controller=PID  Form=Parallel  TimeDomain=Continuous-time  UseExternalTs=off  SampleTime=-1  IntegratorMethod=Forward Euler  FilterMethod=Forward Euler  ControllerParametersSource=internal  P=controllerGains_traction.attitudeRoll_P  I=controllerGains_traction.attitudeRoll_I  UseKiTs=off  D=controllerGains_traction.attitudeRoll_D  UseExternalDerivativeSource=off  N=1  UseFilter=on  TunerSelectOption=Transfer Function Based (PID Tuner App)  InitialConditionSource=internal  InitialConditionForIntegrator=0  InitialConditionForFilter=0  DifferentiatorICPrevScaledInput=0  ExternalReset=rising  TrackingMode=off  Kt=1  LimitOutput=off  SatLimitsSource=internal  UpperSaturationLimit=pi  LowerSaturationLimit=-pi  LinearizeAsGain=on  AntiWindupMode=none  Kb=50  LimitIntegrator=off  UpperIntegratorSaturationLimit=inf  LowerIntegratorSaturationLimit=-inf  POutMin=[]  POutMax=[]  IOutMin=[]  IOutMax=[]  DOutMin=[]  DOutMax=[]  NOutMin=[]  NOutMax=[]  SumOutMin=[]  SumOutMax=[]  SaturationOutMin=[]  SaturationOutMax=[]  PParamMin=[]  PParamMax=[]  IParamMin=[]  IParamMax=[]  DParamMin=[]  DParamMax=[]  NParamMin=[]  NParamMax=[]  KbParamMin=[]  KbParamMax=[]  KtParamMin=[]  KtParamMax=[]  KbOutMin=[]  KbOutMax=[]  KtOutMin=[]  KtOutMax=[]  IntegratorOutMin=[]  IntegratorOutMax=[]  FilterOutMin=[]  FilterOutMax=[]  SumI1OutMin=[]  SumI1OutMax=[]  SumI2OutMin=[]  SumI2OutMax=[]  SumI3OutMin=[]  SumI3OutMax=[]  SumI4OutMin=[]  SumI4OutMax=[]  SumDOutMin=[]  SumDOutMax=[]  DifferentiatorOutMin=[]  DifferentiatorOutMax=[]  FilterDiffOutCoefMin=[]  FilterDiffOutCoefMax=[]  ReciprocalOutMin=[]  ReciprocalOutMax=[]  SumDenOutMin=[]  SumDenOutMax=[]  SumNumOutMin=[]  SumNumOutMax=[]  DivideOutMin=[]  DivideOutMax=[]  UdiffTsProdOutMin=[]  UdiffTsProdOutMax=[]  NTsProdOutMin=[]  NTsProdOutMax=[]  UintegralTsProdOutMin=[]  UintegralTsProdOutMax=[]  UngainTsProdOutMin=[]  UngainTsProdOutMax=[]  ClampingZeroOutDataTypeStr=Inherit: Inherit via back propagation  ClampingZeroOutMin=[]  ClampingZeroOutMax=[]  FilterDenConstantOutDataTypeStr=Inherit: Inherit via back propagation  FilterDenConstantOutMin=[]  FilterDenConstantOutMax=[]  PCopyOutDataTypeStr=Inherit: Inherit via back propagation  PCopyOutMin=[]  PCopyOutMax=[]  NCopyOutDataTypeStr=Inherit: Inherit via back propagation  NCopyOutMin=[]  NCopyOutMax=[]  IntegratorContinuousStateAttributes=''  IntegratorStateMustResolveToSignalObject=off  IntegratorRTWStateStorageClass=Auto  FilterContinuousStateAttributes=''  FilterStateMustResolveToSignalObject=off  FilterRTWStateStorageClass=Auto  ParallelPVariant=InternalParameters  IdealPVariant=Disabled  IVariant=InternalParameters  DVariant=InternalParameters  IntegratorVariant=Continuous  SatVariant=Disabled  AWVariant=Passthrough  PCopyVariant=Disabled  TRVariant=Disabled  FdbkBlocksVariant=Forward  IdealPFdbkVariant=Disabled  SatFdbkVariant=Disabled  DerivativeFilterVariant=ContFilter  NVariant=InternalParameters  NCopyVariant=Disabled  FilterICVariant=InternalICsFilter  IntegratorICVariant=InternalICs  ExternalResetVariant=ExternalReset  TRSumVariant=Passthrough  SumFdbkVariant=Disabled  SumVariant=Sum_PID  TsampFilterVariant=InternalTs  TsampNgainVariant=Passthrough  TsampIntegralVariant=Disabled_SignalSpec  ExternalSaturationOutDataTypeStr=Inherit: Same as second input  DerivativeSourceVariant=ErrorSignal
  PID Controller5 : slpidlib/PID Controller  Controller=PID  Form=Parallel  TimeDomain=Continuous-time  UseExternalTs=off  SampleTime=-1  IntegratorMethod=Forward Euler  FilterMethod=Forward Euler  ControllerParametersSource=internal  P=controllerGains_retraction.attitudeRoll_P  I=controllerGains_retraction.attitudeRoll_I  UseKiTs=off  D=controllerGains_retraction.attitudeRoll_D  UseExternalDerivativeSource=off  N=5  UseFilter=on  TunerSelectOption=Transfer Function Based (PID Tuner App)  InitialConditionSource=internal  InitialConditionForIntegrator=0  InitialConditionForFilter=0  DifferentiatorICPrevScaledInput=0  ExternalReset=rising  TrackingMode=off  Kt=1  LimitOutput=off  SatLimitsSource=internal  UpperSaturationLimit=pi  LowerSaturationLimit=-pi  LinearizeAsGain=on  AntiWindupMode=none  Kb=50  LimitIntegrator=off  UpperIntegratorSaturationLimit=inf  LowerIntegratorSaturationLimit=-inf  POutMin=[]  POutMax=[]  IOutMin=[]  IOutMax=[]  DOutMin=[]  DOutMax=[]  NOutMin=[]  NOutMax=[]  SumOutMin=[]  SumOutMax=[]  SaturationOutMin=[]  SaturationOutMax=[]  PParamMin=[]  PParamMax=[]  IParamMin=[]  IParamMax=[]  DParamMin=[]  DParamMax=[]  NParamMin=[]  NParamMax=[]  KbParamMin=[]  KbParamMax=[]  KtParamMin=[]  KtParamMax=[]  KbOutMin=[]  KbOutMax=[]  KtOutMin=[]  KtOutMax=[]  IntegratorOutMin=[]  IntegratorOutMax=[]  FilterOutMin=[]  FilterOutMax=[]  SumI1OutMin=[]  SumI1OutMax=[]  SumI2OutMin=[]  SumI2OutMax=[]  SumI3OutMin=[]  SumI3OutMax=[]  SumI4OutMin=[]  SumI4OutMax=[]  SumDOutMin=[]  SumDOutMax=[]  DifferentiatorOutMin=[]  DifferentiatorOutMax=[]  FilterDiffOutCoefMin=[]  FilterDiffOutCoefMax=[]  ReciprocalOutMin=[]  ReciprocalOutMax=[]  SumDenOutMin=[]  SumDenOutMax=[]  SumNumOutMin=[]  SumNumOutMax=[]  DivideOutMin=[]  DivideOutMax=[]  UdiffTsProdOutMin=[]  UdiffTsProdOutMax=[]  NTsProdOutMin=[]  NTsProdOutMax=[]  UintegralTsProdOutMin=[]  UintegralTsProdOutMax=[]  UngainTsProdOutMin=[]  UngainTsProdOutMax=[]  ClampingZeroOutDataTypeStr=Inherit: Inherit via back propagation  ClampingZeroOutMin=[]  ClampingZeroOutMax=[]  FilterDenConstantOutDataTypeStr=Inherit: Inherit via back propagation  FilterDenConstantOutMin=[]  FilterDenConstantOutMax=[]  PCopyOutDataTypeStr=Inherit: Inherit via back propagation  PCopyOutMin=[]  PCopyOutMax=[]  NCopyOutDataTypeStr=Inherit: Inherit via back propagation  NCopyOutMin=[]  NCopyOutMax=[]  IntegratorContinuousStateAttributes=''  IntegratorStateMustResolveToSignalObject=off  IntegratorRTWStateStorageClass=Auto  FilterContinuousStateAttributes=''  FilterStateMustResolveToSignalObject=off  FilterRTWStateStorageClass=Auto  ParallelPVariant=InternalParameters  IdealPVariant=Disabled  IVariant=InternalParameters  DVariant=InternalParameters  IntegratorVariant=Continuous  SatVariant=Disabled  AWVariant=Passthrough  PCopyVariant=Disabled  TRVariant=Disabled  FdbkBlocksVariant=Forward  IdealPFdbkVariant=Disabled  SatFdbkVariant=Disabled  DerivativeFilterVariant=ContFilter  NVariant=InternalParameters  NCopyVariant=Disabled  FilterICVariant=InternalICsFilter  IntegratorICVariant=InternalICs  ExternalResetVariant=ExternalReset  TRSumVariant=Passthrough  SumFdbkVariant=Disabled  SumVariant=Sum_PID  TsampFilterVariant=InternalTs  TsampNgainVariant=Passthrough  TsampIntegralVariant=Disabled_SignalSpec  ExternalSaturationOutDataTypeStr=Inherit: Same as second input  DerivativeSourceVariant=ErrorSignal
  Relational Operator2 : RelationalOperator  Operator===  OutDataTypeStr=boolean  RndMeth=Simplest  InputSameDT=off
  Relational Operator3 : RelationalOperator  Operator===  OutDataTypeStr=boolean  RndMeth=Simplest  InputSameDT=off
  Saturation1 : Saturate  UpperLimit=5  LowerLimit=-5
  Scope : Scope
  Sum : Sum  Inputs=|+-
  To Workspace : ToWorkspace  VariableName=Rolldes  SaveFormat=Timeseries  SampleTime=-1
  To Workspace1 : ToWorkspace  VariableName=RollAct  SaveFormat=Timeseries  SampleTime=-1
  To Workspace2 : ToWorkspace  VariableName=RollErr  SaveFormat=Timeseries  SampleTime=-1
  "roll " : Scope  NumInputPorts=3
  desiredRollRate : Outport
  wires:
  Relational Operator3/1 -> PID Controller2/2
  [F_state] -> Scope/1, Multiport Switch2/1
  [F_state] -> Relational Operator3/1, Relational Operator2/1
  PID Controller2/1 -> Multiport Switch2/2
  Sum/1 -> PID Controller5/1, PID Controller2/1, To Workspace2/1, "roll "/3  "roll error"
  desiredRoll/1 -> To Workspace/1, "roll "/1, Sum/1
  Multiport Switch2/1 -> Saturation1/1
  PID Controller5/1 -> Multiport Switch2/4, Multiport Switch2/3
  actualRoll/1 -> Sum/2, To Workspace1/1, "roll "/2
  Relational Operator2/1 -> PID Controller5/2
  Constant3/1 -> Relational Operator3/2
  Constant2/1 -> Relational Operator2/2
  Saturation1/1 -> desiredRollRate/1

== system simL0_multiPath/Controls/AttitudeControl/Yaw ==
  desiredYaw : Inport
  actualYaw : Inport  Port=2
  Constant2 : Constant  Value=2
  Constant3 : Constant
  Multiport Switch2 : MultiPortSwitch  DiagnosticForDefault=None  SaturateOnIntegerOverflow=off  InputSameDT=off
  PID Controller2 : simulink/Continuous/PID Controller  Controller=PI  Form=Parallel  TimeDomain=Continuous-time  SampleTime=-1  IntegratorMethod=Forward Euler  FilterMethod=Forward Euler  ControllerParametersSource=internal  P=controllerGains_traction.attitudeYaw_P  I=controllerGains_traction.attitudeYaw_I  D=controllerGains_traction.attitudeRoll_D  UseFilter=on  N=1  TunerSelectOption=Transfer Function Based (PID Tuner App)  InitialConditionSource=internal  InitialConditionForIntegrator=0  InitialConditionForFilter=0  DifferentiatorICPrevScaledInput=0  ExternalReset=rising  TrackingMode=off  Kt=1  LimitOutput=off  UpperSaturationLimit=pi  LowerSaturationLimit=-pi  LinearizeAsGain=on  AntiWindupMode=none  Kb=50  POutMin=[]  POutMax=[]  IOutMin=[]  IOutMax=[]  DOutMin=[]  DOutMax=[]  NOutMin=[]  NOutMax=[]  SumOutMin=[]  SumOutMax=[]  SaturationOutMin=[]  SaturationOutMax=[]  PParamMin=[]  PParamMax=[]  IParamMin=[]  IParamMax=[]  DParamMin=[]  DParamMax=[]  NParamMin=[]  NParamMax=[]  KbParamMin=[]  KbParamMax=[]  KtParamMin=[]  KtParamMax=[]  KbOutMin=[]  KbOutMax=[]  KtOutMin=[]  KtOutMax=[]  IntegratorOutMin=[]  IntegratorOutMax=[]  FilterOutMin=[]  FilterOutMax=[]  SumI1OutMin=[]  SumI1OutMax=[]  SumI2OutMin=[]  SumI2OutMax=[]  SumI3OutMin=[]  SumI3OutMax=[]  SumI4OutMin=[]  SumI4OutMax=[]  SumDOutMin=[]  SumDOutMax=[]  DifferentiatorOutMin=[]  DifferentiatorOutMax=[]  FilterDiffOutCoefMin=[]  FilterDiffOutCoefMax=[]  ReciprocalOutMin=[]  ReciprocalOutMax=[]  SumDenOutMin=[]  SumDenOutMax=[]  SumNumOutMin=[]  SumNumOutMax=[]  DivideOutMin=[]  DivideOutMax=[]  IntegratorContinuousStateAttributes=''  IntegratorStateMustResolveToSignalObject=off  IntegratorRTWStateStorageClass=Auto  FilterContinuousStateAttributes=''  FilterStateMustResolveToSignalObject=off  FilterRTWStateStorageClass=Auto  ParallelPVariant=InternalParameters  IdealPVariant=Disabled  IVariant=InternalParameters  DVariant=Disabled  IntegratorVariant=Continuous  SatVariant=Disabled  AWVariant=Passthrough  PCopyVariant=Disabled  TRVariant=Disabled  FdbkBlocksVariant=Forward  IdealPFdbkVariant=Disabled  SatFdbkVariant=Disabled  DerivativeFilterVariant=Disabled  NVariant=Disabled  NCopyVariant=Disabled_SignalSpec  FilterICVariant=Disabled  IntegratorICVariant=InternalICs  ExternalResetVariant=ExternalReset  TRSumVariant=Passthrough  SumFdbkVariant=Disabled  SumVariant=Sum_PI
  PID Controller5 : simulink/Continuous/PID Controller  Controller=PI  Form=Parallel  TimeDomain=Continuous-time  SampleTime=-1  IntegratorMethod=Forward Euler  FilterMethod=Forward Euler  ControllerParametersSource=internal  P=controllerGains_retraction.attitudeYaw_P  I=controllerGains_retraction.attitudeYaw_I  D=controllerGains_retraction.attitudeRoll_D  UseFilter=on  N=5  TunerSelectOption=Transfer Function Based (PID Tuner App)  InitialConditionSource=internal  InitialConditionForIntegrator=0  InitialConditionForFilter=0  DifferentiatorICPrevScaledInput=0  ExternalReset=rising  TrackingMode=off  Kt=1  LimitOutput=off  UpperSaturationLimit=pi  LowerSaturationLimit=-pi  LinearizeAsGain=on  AntiWindupMode=none  Kb=50  POutMin=[]  POutMax=[]  IOutMin=[]  IOutMax=[]  DOutMin=[]  DOutMax=[]  NOutMin=[]  NOutMax=[]  SumOutMin=[]  SumOutMax=[]  SaturationOutMin=[]  SaturationOutMax=[]  PParamMin=[]  PParamMax=[]  IParamMin=[]  IParamMax=[]  DParamMin=[]  DParamMax=[]  NParamMin=[]  NParamMax=[]  KbParamMin=[]  KbParamMax=[]  KtParamMin=[]  KtParamMax=[]  KbOutMin=[]  KbOutMax=[]  KtOutMin=[]  KtOutMax=[]  IntegratorOutMin=[]  IntegratorOutMax=[]  FilterOutMin=[]  FilterOutMax=[]  SumI1OutMin=[]  SumI1OutMax=[]  SumI2OutMin=[]  SumI2OutMax=[]  SumI3OutMin=[]  SumI3OutMax=[]  SumI4OutMin=[]  SumI4OutMax=[]  SumDOutMin=[]  SumDOutMax=[]  DifferentiatorOutMin=[]  DifferentiatorOutMax=[]  FilterDiffOutCoefMin=[]  FilterDiffOutCoefMax=[]  ReciprocalOutMin=[]  ReciprocalOutMax=[]  SumDenOutMin=[]  SumDenOutMax=[]  SumNumOutMin=[]  SumNumOutMax=[]  DivideOutMin=[]  DivideOutMax=[]  IntegratorContinuousStateAttributes=''  IntegratorStateMustResolveToSignalObject=off  IntegratorRTWStateStorageClass=Auto  FilterContinuousStateAttributes=''  FilterStateMustResolveToSignalObject=off  FilterRTWStateStorageClass=Auto  ParallelPVariant=InternalParameters  IdealPVariant=Disabled  IVariant=InternalParameters  DVariant=Disabled  IntegratorVariant=Continuous  SatVariant=Disabled  AWVariant=Passthrough  PCopyVariant=Disabled  TRVariant=Disabled  FdbkBlocksVariant=Forward  IdealPFdbkVariant=Disabled  SatFdbkVariant=Disabled  DerivativeFilterVariant=Disabled  NVariant=Disabled  NCopyVariant=Disabled_SignalSpec  FilterICVariant=Disabled  IntegratorICVariant=InternalICs  ExternalResetVariant=ExternalReset  TRSumVariant=Passthrough  SumFdbkVariant=Disabled  SumVariant=Sum_PI
  Relational Operator2 : RelationalOperator  OutDataTypeStr=boolean  RndMeth=Simplest  InputSameDT=off
  Relational Operator3 : RelationalOperator  Operator===  OutDataTypeStr=boolean  RndMeth=Simplest  InputSameDT=off
  Scope : Scope  NumInputPorts=2
  Sum : Sum  Inputs=|+-
  To Workspace : ToWorkspace  VariableName=Yawdes  SaveFormat=Timeseries  SampleTime=-1
  To Workspace1 : ToWorkspace  VariableName=YawAct  SaveFormat=Timeseries  SampleTime=-1
  To Workspace2 : ToWorkspace  VariableName=YawErr  SaveFormat=Timeseries  SampleTime=-1
  "yaw " : Scope  NumInputPorts=3
  desiredyawRate : Outport
  wires:
  Relational Operator3/1 -> PID Controller2/2
  [F_state] -> Multiport Switch2/1
  [F_state] -> Relational Operator3/1, Relational Operator2/1
  PID Controller2/1 -> Scope/1, Multiport Switch2/2
  Sum/1 -> PID Controller5/1, PID Controller2/1, To Workspace2/1, "yaw "/3  "yaw error"
  desiredYaw/1 -> To Workspace/1, "yaw "/1, Sum/1
  PID Controller5/1 -> Multiport Switch2/4, Multiport Switch2/3
  actualYaw/1 -> Sum/2, To Workspace1/1, "yaw "/2
  Relational Operator2/1 -> PID Controller5/2
  Constant3/1 -> Relational Operator3/2
  Constant2/1 -> Relational Operator2/2
  Multiport Switch2/1 -> Scope/2, desiredyawRate/1

== system simL0_multiPath/Controls/RatesControl/rate controller ==
  p_c : Inport
  q_c : Inport  Port=2
  r_c : Inport  Port=3
  p : Inport  Port=4
  q : Inport  Port=5
  r : Inport  Port=6
  V_T : Inport  Port=7
  From : From  Commented=on  GotoTag=vel_squared
  Pitch : Subsystem
  "Roll " : Subsystem
  Scope : Scope  NumInputPorts=3
  Scope1 : Scope  NumInputPorts=3
  Sum : Sum  Inputs=|+-
  Sum1 : Sum  Inputs=|+-
  Sum2 : Sum  Commented=on  Inputs=|+-
  Yaw : Subsystem  Commented=on
  squared Function : Math  Operator=square  SignedPower=on
  roll : Outport  VectorParamsAs1DForOutWhenUnconnected=off
  pitch : Outport  Port=2  VectorParamsAs1DForOutWhenUnconnected=off
  yaw : Outport  Port=3  VectorParamsAs1DForOutWhenUnconnected=off
  wires:
  r_c/1 -> Sum2/1
  q_c/1 -> Scope/2, Sum1/1
  p/1 -> Scope1/2, Sum/2  "r_rate"
  q/1 -> Scope/3, Sum1/2
  r/1 -> Sum2/2
  V_T/1 -> squared Function/1
  Sum1/1 -> Scope/1, Pitch/1(In1)  "pitch"
  Pitch/1(Out1) -> pitch/1
  Sum/1 -> Scope1/3, "Roll "/1(In1)  "r_rate_err"
  "Roll "/1(Out1) -> roll/1
  Yaw/1(Out1) -> yaw/1
  Sum2/1 -> Yaw/1(In1)  "yaw"
  squared Function/1 -> [vel_squared]  "V_T"
  From/1 -> Yaw/2(In2)
  [vel_squared] -> "Roll "/2(In2)
  [vel_squared] -> Pitch/2(In2)
  p_c/1 -> Scope1/1, Sum/1  "r_rate des"

== system simL0_multiPath/GroundStationMegAWES/Traction winch controller/Calculate Ft_ref ==
  v_ro : Inport
  Zgraggen tether force reference : MATLAB Function  TreatAsAtomicUnit=on
  Ft_ref : Outport
  wires:
  Zgraggen tether force reference/1(Ft_ref) -> Ft_ref/1
  v_ro/1 -> Zgraggen tether force reference/1(v_ro)

== system simL0_multiPath/Controls/ FlightControl/traction/EarthtoWind2 ==
  E_vec : Inport
  Demux : Demux  Outputs=3
  Gain : Gain
  Gain1 : Gain  Gain=-1
  Gain2 : Gain  Gain=-1
  Mux4 : Mux  Inputs=3
  W_vec : Outport
  wires:
  Demux/2 -> Gain1/1
  Demux/1 -> Gain/1
  Gain1/1 -> Mux4/2
  Gain/1 -> Mux4/1
  Gain2/1 -> Mux4/3
  E_vec/1 -> Demux/1
  Mux4/1 -> W_vec/1
  Demux/3 -> Gain2/1

== system simL0_multiPath/Controls/ FlightControl/traction/EarthtoWind3 ==
  E_vec : Inport
  Demux : Demux  Outputs=3
  Gain : Gain
  Gain1 : Gain  Gain=-1
  Gain2 : Gain  Gain=-1
  Mux4 : Mux  Inputs=3
  W_vec : Outport
  wires:
  Demux/2 -> Gain1/1
  Demux/1 -> Gain/1
  Gain1/1 -> Mux4/2
  Gain/1 -> Mux4/1
  Gain2/1 -> Mux4/3
  E_vec/1 -> Demux/1
  Mux4/1 -> W_vec/1
  Demux/3 -> Gain2/1
